simulink model "figure_1_11"  (R2026a)
settings: Solver=ode5  FixedStep=1e-4
settings Model: Creator=yagmu  LastModifiedBy=yagmu

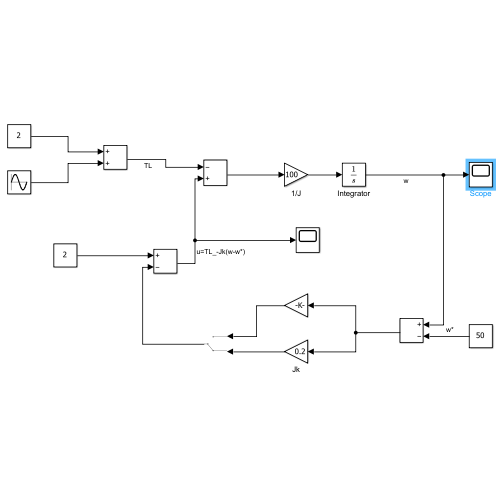
[thumbnail: Simulink's stored preview of the top-level diagram]
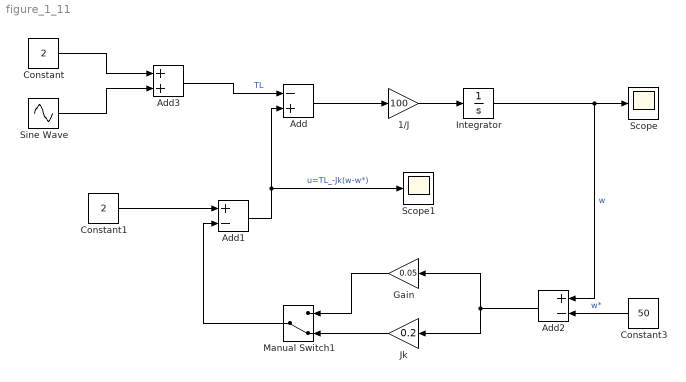
== system figure_1_11 ==
  1/J : Gain  Gain=100
  Add : Sum  Inputs=-+
  Add1 : Sum  Inputs=+-
  Add2 : Sum  Inputs=+-
  Add3 : Sum
  Constant : Constant  Value=2
  Constant1 : Constant  Value=2
  Constant3 : Constant  Value=50
  Gain : Gain  Gain=0.05
  Integrator : Integrator  InitialCondition=50
  Jk : Gain  Gain=0.2
  Manual Switch1 : ManualSwitch  CurrentSetting=0
  Scope : Scope
      settings: ActiveDisplayYMinimum=48.913098206795333  ActiveDisplayYMaximum=51.073536773490282
  Scope1 : Scope
      settings: ActiveDisplayYMinimum=1.7852926453019433  ActiveDisplayYMaximum=2.2173803586409342
  Sine Wave : Sin  Amplitude=0.2  Frequency=12  SampleTime=0
  wires:
  Add/1 -> 1/J/1
  1/J/1 -> Integrator/1
  Integrator/1 -> Add2/1, Scope/1  "w"
  Add1/1 -> Add/2, Scope1/1  "u=TL_-Jk(w-w*)"
  Manual Switch1/1 -> Add1/2
  Constant3/1 -> Add2/2  "w*"
  Gain/1 -> Manual Switch1/1
  Jk/1 -> Manual Switch1/2
  Add2/1 -> Jk/1, Gain/1
  Constant1/1 -> Add1/1
  Constant/1 -> Add3/1
  Sine Wave/1 -> Add3/2
  Add3/1 -> Add/1  "TL"
